simulink model "visualization_model"  (R2025a)
settings: Solver=VariableStepAuto  StartTime=0.0  StopTime=inf  RelTol=1e-3
libraries: sim3dlib x2
settings Model: Creator=brzan  LastModifiedBy=brzan

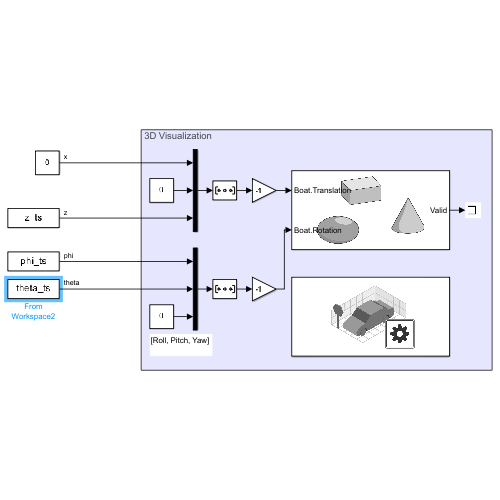
[thumbnail: Simulink's stored preview of the top-level diagram]
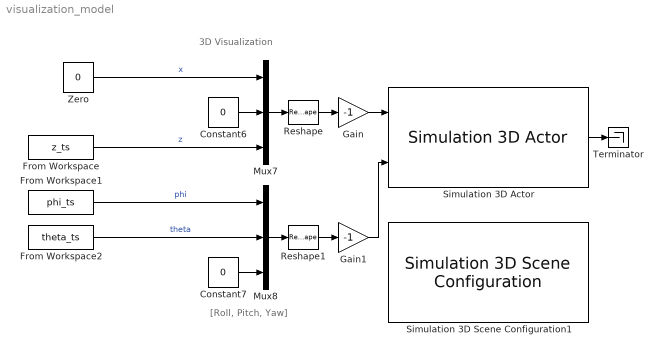
== system visualization_model ==
  note: 3D Visualization
  note: [Roll, Pitch, Yaw]
  Constant6 : Constant  Value=0
  Constant7 : Constant  Value=0
  From Workspace : FromWorkspace  VariableName=z_ts  OutputAfterFinalValue=Holding final value
  From Workspace1 : FromWorkspace  VariableName=phi_ts  OutputAfterFinalValue=Holding final value
  From Workspace2 : FromWorkspace  VariableName=theta_ts  OutputAfterFinalValue=Holding final value
  Gain : Gain  Gain=-1
  Gain1 : Gain  Gain=-1
  Mux7 : Mux  Inputs=3
  Mux8 : Mux  Inputs=3
  Reshape : Reshape  OutputDimensionality=Row vector (2-D)
  Reshape1 : Reshape  OutputDimensionality=Row vector (2-D)
  Simulation 3D Actor : sim3dlib/Simulation 3D Actor  Priority=1  ActorName=Boat  ParentName=Scene Origin  Operation=Create at setup  InitScriptText=|  SampleTime=-1  Translation=[0 0 0]  Rotation=[0 0 0]  Scale=[1 1 1]/1000  InputsText=Boat.Translation Boat.Rotation  aMode=5  ActorTag=Boat  ActorType=Sim3dActor  ID=C
      | % Reserved keywords:
      | % - Actor : handle to this actor object
      | % - World : handle to the world object
      | 
      | % Examples:
      | 
      | % Create a primitive geometry (optional)
      | % createShape(Actor, 'box', [1 1 1]);
      | 
      | % Initialize values (optional)
      | % Actor.Physics = true;
      | % Actor.Color = [1 0 0];
  Simulation 3D Scene Configuration1 : sim3dlib/Simulation 3D Scene Configuration  Priority=0  ProjectFormat=Default Scenes  SceneDesc=Open surface  ProjectName=C:\Program Files\MATLAB\R2025a\toolbox\shared\sim3d_projects\automotive_project_windows\UE\WindowsNoEditor\VehicleSimulation.exe  ScenePath=/Game/Maps/HwStrght  EnableOpenDRIVE=off  vehTagList={'Boat';'Custom';'Scene Origin'}  vehTag=Boat  AttachedCameraRelativeTranslation=[-4 -3 1]*1000*0.25  FreeCameraDefaultInitialTranslation=[-6, 0, 2]  AttachedCameraRelativeRotation=[0 -10 40]  FreeCameraDefaultInitialRotation=[0, -15, 0]  ViewpointName=Custom  FreeCameraInitialTranslation=[-5 0 1]  ViewpointTranslation=[0 0 0]  FreeCameraInitialRotation=[0 0 0]  ViewpointRotation=[0 0 0]  OpVisEn=off  Ts=.05  EnableWindow=on  EnableRemoteAccess=off  EnableWeather=off  SunAzimuth=90  SunAltitude=40.0  EnableGeospatialSun=off  Latitude=0  Longitude=0  Date=2023-01-01  Time=10:30:00  GeoTimeZone=-5.0  SunDaylightSaving=off  wind=1  clouds=10  EnableVolumetricClouds=off  CloudCoverage=0  CloudAltitude=6  fog=0  rain=0  RaindropsEffect=off  SnowDensity=0  EnableGeospatial=off  TilesetSource=Earth terrain  UseTrueOrigin=off  OriginHeight=200  OriginLatitude=40.744652  OriginLongitude=-73.988864  MapStyle=Aerial  AdditionalAssetIDs=[]  UseAdvancedSunSky=off  SolarTime=11  TimeZone=-5  Day=21  Month=9  Year=2022  UseDaylightSavingTime=on  DSTStartDay=10  DSTStartMonth=3  DSTEndDay=3  DSTEndMonth=11  DSTSwitchHour=2  sensorTag=MainCamera1  sensorId=1  sensorName=MainCamera1  mountLoc=Origin  offsetFlag=off  tmountOffset=[0, 0, 0]  rmountOffset=[0, 0, 0]  HorizontalResolution=1280  VerticalResolution=720  HorizontalFOV=60  mountPoint=[0 0 0]  mountOrientation=[0 0 0]  aMode=5  ID=1  GeoTrigger=Inactive  ViewNameList={'Custom'}  ViewTranslationList={'[-5 0 1]'}  ViewRotationList={'[0 0 0]'}
      settings: LibrarySourceBlock=sl3dlib/Simulation 3D/Environment/Simulation 3D Scene Configuration
  Terminator : Terminator
  Zero : Constant  Value=0  OutDataTypeStr=Inherit: Inherit via back propagation
  wires:
  Mux7/1 -> Reshape/1
  From Workspace2/1 -> Mux8/2  "theta"
  Reshape/1 -> Gain/1
  Constant7/1 -> Mux8/3
  From Workspace1/1 -> Mux8/1  "phi"
  Mux8/1 -> Reshape1/1
  Constant6/1 -> Mux7/2
  Simulation 3D Actor/1 -> Terminator/1
  Reshape1/1 -> Gain1/1
  Gain/1 -> Simulation 3D Actor/1
  From Workspace/1 -> Mux7/3  "z"
  Gain1/1 -> Simulation 3D Actor/2
  Zero/1 -> Mux7/1  "x"
